simulink model "TestMotorMap"  (R2018b)
settings: Solver=VariableStepAuto  StartTime=0.0  StopTime=10.0  RelTol=1e-3
settings Model: Creator=jban039  LastModifiedBy=jban039

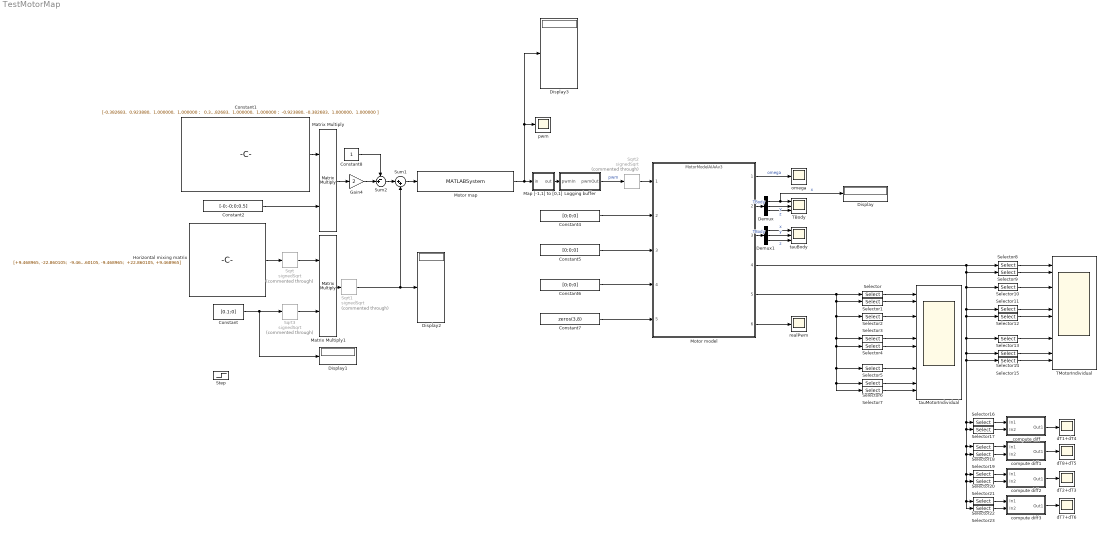
== system TestMotorMap ==
  Constant : Constant  Value=[0.1;0]
  Constant1 : Constant  Value=|
      | [-0.382683,  0.923880,  1.000000,  1.000000 ;
      |   0.382683, -0.923880,  1.000000,  1.000000 ;
      |  -0.923880,  0.382683, -1.000000,  1.000000 ;
      |  -0.382683, -0.923880, -1.000000,  1.000000 ;
      |   0.382683,  0.923880, -1.000000,  1.000000 ;
      |   0.923880, -0.382683, -1.000000,  1.000000 ;
      |   0.923880,  0.382683,  1.000000,  1.000000 ;
      |  -0.923880, -0.382683,  1.000000,  1.000000 ]
  Constant2 : Constant  Value=[-0;-0;0;0.5]
  Constant4 : Constant  Value=[0;0;0]
  Constant5 : Constant  Value=[0;0;0]
  Constant6 : Constant  Value=[0;0;0]
  Constant7 : Constant  Value=zeros(3,8)
  Constant8 : Constant
  Demux : Demux  Outputs=3
  Demux1 : Demux  Outputs=3
  Display{,1..3} (4 alike) : Display
  Gain4 : Gain  Gain=2
  Horizontal mixing matrix : Constant  Value=|
      | [+9.468965, -22.860105;
      |  -9.468965, +22.860105;
      |  -22.860105, +9.468965;
      |  -9.468965, -22.860105;
      |  +9.468965, +22.860105;
      |  +22.860105, -9.468965;
      |  -22.860105, -9.468965;
      |  +22.860105, +9.468965]
  Logging buffer : Subsystem
  Map [-1,1] to [0,1] : Subsystem
  Matrix Multiply : Product  Multiplication=Matrix(*)
  Matrix Multiply1 : Product  Multiplication=Matrix(*)
  Motor map : MATLABSystem  System=MotorMap  airframeConfig=5  SimulateUsing=Code generation
      mask Type: MotorMap
      mask Display:
      | disp(['MOTOR' char(10) 'MAP' char(10) 'octa_x']);
      | port_label('input',1,'px4PWM');
      | port_label('output',1,'simPWM');
  Motor model : ModelReference  ModelNameDialog=MotorModelAIAAv3  SimulationMode=Normal  ModelReferenceVersion=1.397
  Selector : Selector  NumberOfDimensions=2  InputPortWidth=[8,3]  IndexOptions=Select all,Index vector (dialog)  Indices=3,7  OutputSizes=1,1
  Selector1 : Selector  NumberOfDimensions=2  InputPortWidth=[8,3]  IndexOptions=Select all,Index vector (dialog)  Indices=3,6  OutputSizes=1,1
  Selector10 : Selector  NumberOfDimensions=2  InputPortWidth=[8,3]  IndexOptions=Select all,Index vector (dialog)  Indices=3,8  OutputSizes=1,1
  Selector11 : Selector  NumberOfDimensions=2  InputPortWidth=[8,3]  IndexOptions=Select all,Index vector (dialog)  Indices=3,5  OutputSizes=1,1
  Selector12 : Selector  NumberOfDimensions=2  InputPortWidth=[8,3]  IndexOptions=Select all,Index vector (dialog)  Indices=3,1  OutputSizes=1,1
  Selector13 : Selector  NumberOfDimensions=2  InputPortWidth=[8,3]  IndexOptions=Select all,Index vector (dialog)  Indices=3,4  OutputSizes=1,1
  Selector14 : Selector  NumberOfDimensions=2  InputPortWidth=[8,3]  IndexOptions=Select all,Index vector (dialog)  Indices=3,2  OutputSizes=1,1
  Selector15 : Selector  NumberOfDimensions=2  InputPortWidth=[8,3]  IndexOptions=Select all,Index vector (dialog)  Indices=3,3  OutputSizes=1,1
  Selector16 : Selector  NumberOfDimensions=2  InputPortWidth=[8,3]  IndexOptions=Index vector (dialog),Index vector (dialog)  Indices=3,1  OutputSizes=1,1
  Selector17 : Selector  NumberOfDimensions=2  InputPortWidth=[8,3]  IndexOptions=Index vector (dialog),Index vector (dialog)  Indices=3,4  OutputSizes=1,1
  Selector18 : Selector  NumberOfDimensions=2  InputPortWidth=[8,3]  IndexOptions=Index vector (dialog),Index vector (dialog)  Indices=3,8  OutputSizes=1,1
  Selector19 : Selector  NumberOfDimensions=2  InputPortWidth=[8,3]  IndexOptions=Index vector (dialog),Index vector (dialog)  Indices=3,5  OutputSizes=1,1
  Selector2 : Selector  NumberOfDimensions=2  InputPortWidth=[8,3]  IndexOptions=Select all,Index vector (dialog)  Indices=3,8  OutputSizes=1,1
  Selector20 : Selector  NumberOfDimensions=2  InputPortWidth=[8,3]  IndexOptions=Index vector (dialog),Index vector (dialog)  Indices=3,2  OutputSizes=1,1
  Selector21 : Selector  NumberOfDimensions=2  InputPortWidth=[8,3]  IndexOptions=Index vector (dialog),Index vector (dialog)  Indices=3,3  OutputSizes=1,1
  Selector22 : Selector  NumberOfDimensions=2  InputPortWidth=[8,3]  IndexOptions=Index vector (dialog),Index vector (dialog)  Indices=3,7  OutputSizes=1,1
  Selector23 : Selector  NumberOfDimensions=2  InputPortWidth=[8,3]  IndexOptions=Index vector (dialog),Index vector (dialog)  Indices=3,6  OutputSizes=1,1
  Selector3 : Selector  NumberOfDimensions=2  InputPortWidth=[8,3]  IndexOptions=Select all,Index vector (dialog)  Indices=3,5  OutputSizes=1,1
  Selector4 : Selector  NumberOfDimensions=2  InputPortWidth=[8,3]  IndexOptions=Select all,Index vector (dialog)  Indices=3,1  OutputSizes=1,1
  Selector5 : Selector  NumberOfDimensions=2  InputPortWidth=[8,3]  IndexOptions=Select all,Index vector (dialog)  Indices=3,4  OutputSizes=1,1
  Selector6 : Selector  NumberOfDimensions=2  InputPortWidth=[8,3]  IndexOptions=Select all,Index vector (dialog)  Indices=3,2  OutputSizes=1,1
  Selector7 : Selector  NumberOfDimensions=2  InputPortWidth=[8,3]  IndexOptions=Select all,Index vector (dialog)  Indices=3,3  OutputSizes=1,1
  Selector8 : Selector  NumberOfDimensions=2  InputPortWidth=[8,3]  IndexOptions=Select all,Index vector (dialog)  Indices=3,7  OutputSizes=1,1
  Selector9 : Selector  NumberOfDimensions=2  InputPortWidth=[8,3]  IndexOptions=Select all,Index vector (dialog)  Indices=3,6  OutputSizes=1,1
  Sqrt{,1..3} (4 alike) : Sqrt  Commented=through  Operator=signedSqrt  SaturateOnIntegerOverflow=on
  Step : Step  Time=5  Before=[0;0]  After=[0.01;0]  SampleTime=0
  Sum1 : Sum  Inputs=|++
  Sum2 : Sum  Inputs=-+|
  TBody : Scope  NumInputPorts=3
  TMotorIndividual : Scope  NumInputPorts=16
  compute diff : Subsystem
  compute diff1 : Subsystem
  compute diff2 : Subsystem
  compute diff3 : Subsystem
  dT1+dT4 : Scope
  dT2+dT3 : Scope
  dT7+dT6 : Scope
  dT8+dT5 : Scope
  omega : Scope
  pwm : Scope
  realPwm : Scope
  tauBody : Scope  NumInputPorts=3
  tauMotorIndividual : Scope  NumInputPorts=16
  wires:
  Map [-1,1] to [0,1]/1(out) -> Logging buffer/1(pwmIn)
  Motor map/1 -> Display3/1, pwm/1, Map [-1,1] to [0,1]/1(in)
  Logging buffer/1(pwmOut) -> Sqrt2/1  "pwm"
  Constant/1 -> Display1/1, Sqrt3/1
  Horizontal mixing matrix/1 -> Sqrt/1
  Matrix Multiply1/1 -> Sqrt1/1
  Gain4/1 -> Sum2/2
  Sum2/1 -> Sum1/1
  Constant1/1 -> Matrix Multiply/1
  Constant2/1 -> Matrix Multiply/2
  Constant4/1 -> Motor model/2
  Constant5/1 -> Motor model/3
  Constant6/1 -> Motor model/4
  Constant7/1 -> Motor model/5
  Motor model/5 -> Selector7/1, Selector6/1, Selector5/1, Selector4/1, Selector3/1, Selector2/1, Selector1/1, Selector/1
  Motor model/6 -> realPwm/1
  Motor model/2 -> Demux/1  "TBody"
  Demux/1 -> Display/1, TBody/1  "x"
  Demux/2 -> TBody/2  "y"
  Demux/3 -> TBody/3  "z"
  Demux1/3 -> tauBody/3  "z"
  Demux1/2 -> tauBody/2  "y"
  Demux1/1 -> tauBody/1  "x"
  Motor model/3 -> Demux1/1  "TBody"
  Motor model/1 -> omega/1  "omega"
  Constant8/1 -> Sum2/1
  Selector/1 -> tauMotorIndividual/2
  Selector1/1 -> tauMotorIndividual/3
  Selector2/1 -> tauMotorIndividual/5
  Selector3/1 -> tauMotorIndividual/8
  Selector4/1 -> tauMotorIndividual/9
  Selector5/1 -> tauMotorIndividual/12
  Selector7/1 -> tauMotorIndividual/15
  Selector6/1 -> tauMotorIndividual/14
  Selector14/1 -> TMotorIndividual/14
  Selector15/1 -> TMotorIndividual/15
  Selector13/1 -> TMotorIndividual/12
  Selector12/1 -> TMotorIndividual/9
  Selector11/1 -> TMotorIndividual/8
  Selector10/1 -> TMotorIndividual/5
  Selector9/1 -> TMotorIndividual/3
  Selector8/1 -> TMotorIndividual/2
  Motor model/4 -> Selector8/1, Selector9/1, Selector10/1, Selector11/1, Selector12/1, Selector13/1, Selector14/1, Selector23/1, Selector22/1, Selector21/1, Selector20/1, Selector19/1, Selector18/1, Selector17/1, Selector16/1, Selector15/1
  Sqrt/1 -> Matrix Multiply1/1
  Selector16/1 -> compute diff/1(In1)
  Selector17/1 -> compute diff/2(In2)
  compute diff/1(Out1) -> dT1+dT4/1
  compute diff1/1(Out1) -> dT8+dT5/1
  Selector19/1 -> compute diff1/2(In2)
  Selector18/1 -> compute diff1/1(In1)
  Selector20/1 -> compute diff2/1(In1)
  Selector21/1 -> compute diff2/2(In2)
  compute diff2/1(Out1) -> dT2+dT3/1
  compute diff3/1(Out1) -> dT7+dT6/1
  Selector23/1 -> compute diff3/2(In2)
  Selector22/1 -> compute diff3/1(In1)
  Sqrt1/1 -> Display2/1, Sum1/2
  Sqrt2/1 -> Motor model/1
  Sqrt3/1 -> Matrix Multiply1/2
  Matrix Multiply/1 -> Gain4/1
  Sum1/1 -> Motor map/1

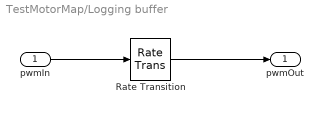
== system TestMotorMap/Logging buffer ==
  pwmIn : Inport
  Rate Transition : RateTransition  SCDEnableBlockLinearizationSpecification=on
  pwmOut : Outport
  wires:
  Rate Transition/1 -> pwmOut/1
  pwmIn/1 -> Rate Transition/1

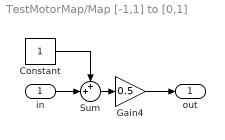
== system TestMotorMap/Map [-1,1] to [0,1] ==
  in : Inport
  Constant : Constant
  Gain4 : Gain  Gain=0.5
  Sum : Sum  Inputs=++|
  out : Outport
  wires:
  Constant/1 -> Sum/1
  in/1 -> Sum/2
  Gain4/1 -> out/1
  Sum/1 -> Gain4/1

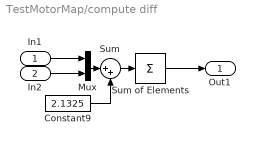
== system TestMotorMap/compute diff ==
  In1 : Inport
  In2 : Inport  Port=2
  Constant9 : Constant  Value=2.1325
  Mux : Mux  Inputs=2
  Sum : Sum  Inputs=|++
  Sum of Elements : Sum  Inputs=+
  Out1 : Outport
  wires:
  Sum of Elements/1 -> Out1/1
  Sum/1 -> Sum of Elements/1
  In2/1 -> Mux/2
  Constant9/1 -> Sum/2
  In1/1 -> Mux/1
  Mux/1 -> Sum/1

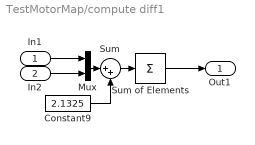
== system TestMotorMap/compute diff1 ==
  In1 : Inport
  In2 : Inport  Port=2
  Constant9 : Constant  Value=2.1325
  Mux : Mux  Inputs=2
  Sum : Sum  Inputs=|++
  Sum of Elements : Sum  Inputs=+
  Out1 : Outport
  wires:
  Mux/1 -> Sum/1
  In1/1 -> Mux/1
  Constant9/1 -> Sum/2
  In2/1 -> Mux/2
  Sum/1 -> Sum of Elements/1
  Sum of Elements/1 -> Out1/1

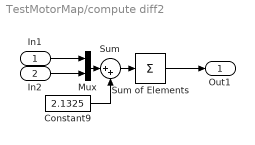
== system TestMotorMap/compute diff2 ==
  In1 : Inport
  In2 : Inport  Port=2
  Constant9 : Constant  Value=2.1325
  Mux : Mux  Inputs=2
  Sum : Sum  Inputs=|++
  Sum of Elements : Sum  Inputs=+
  Out1 : Outport
  wires:
  Sum of Elements/1 -> Out1/1
  Sum/1 -> Sum of Elements/1
  In2/1 -> Mux/2
  Constant9/1 -> Sum/2
  In1/1 -> Mux/1
  Mux/1 -> Sum/1

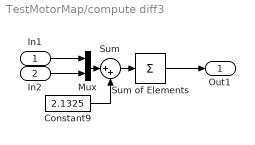
== system TestMotorMap/compute diff3 ==
  In1 : Inport
  In2 : Inport  Port=2
  Constant9 : Constant  Value=2.1325
  Mux : Mux  Inputs=2
  Sum : Sum  Inputs=|++
  Sum of Elements : Sum  Inputs=+
  Out1 : Outport
  wires:
  Mux/1 -> Sum/1
  In1/1 -> Mux/1
  Constant9/1 -> Sum/2
  In2/1 -> Mux/2
  Sum/1 -> Sum of Elements/1
  Sum of Elements/1 -> Out1/1
